simulink model "test5_diff"  (R2017b)
settings: Solver=VariableStepAuto  StartTime=0.0  StopTime=10.0  RelTol=1e-3
settings Model: Creator=monika  LastModifiedBy=monika

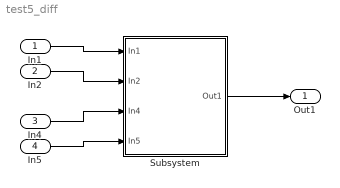
== system test5_diff ==
  In1 : Inport
  In2 : Inport  Port=2
  In4 : Inport  Port=3
  In5 : Inport  Port=4
  Subsystem : Subsystem
  Out1 : Outport
  wires:
  In1/1 -> Subsystem/1(In1)
  Subsystem/1(Out1) -> Out1/1
  In2/1 -> Subsystem/2(In2)
  In4/1 -> Subsystem/3(In4)
  In5/1 -> Subsystem/4(In5)

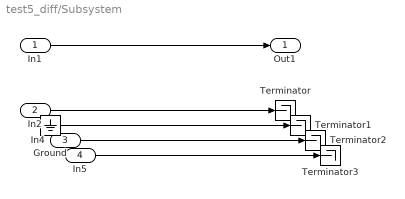
== system test5_diff/Subsystem ==
  In1 : Inport
  In2 : Inport  Port=2
  In4 : Inport  Port=3
  In5 : Inport  Port=4
  Ground : Ground
  Terminator{,1..3} (4 alike) : Terminator
  Out1 : Outport
  wires:
  In1/1 -> Out1/1
  In2/1 -> Terminator/1
  Ground/1 -> Terminator1/1
  In4/1 -> Terminator2/1
  In5/1 -> Terminator3/1
